simulink model "ravvenController"  (R2018b)
settings: Solver=FixedStepAuto  StartTime=0.0  StopTime=inf  FixedStep=1/1000  RelTol=1e-3  EnableMultiTasking=on
values from neighbouring files (symbols this model uses):
  fs = 1000    [setup.m]
  Ka = [ 4  4   2 ]    [setup.m]
  Kcfa = 0.01    [setup.m]
  Kcfw = 0.99    [setup.m]
  Khd = .3    (= 0.3)    [setup.m]
  Kmixing = [  1   1   1  -1 ... (first row only)    [setup.m]
  Kw = [ .01   .01    .2  ]    [setup.m]
  UseSmallAngleApprox = 0    [setup.m]
  UseTrueThetaPhi = 0    [setup.m]
  w_cmd_lim = 200    [setup.m]
libraries: simulink x6
settings Model: SimulationMode=external  TunableVars=Ka,Kpos,Kvel,Kw  TunableVarsStorageClass=Auto,Auto,Auto,Auto  TunableVarsTypeQualifier=,,,  Creator=kowens  LastModifiedBy=axk1188
settings SolverCC: PositivePriorityOrder=on  AutoInsertRateTranBlk=on
settings DataIOCC: LimitDataPoints=on  SaveFormat=Array  SignalLoggingSaveFormat=ModelDataLogs
settings OptimizationCC: PassReuseOutputArgsAs=Individual arguments  ExpressionDepthLimit=2147483647  MaxStackSize=64
settings DebuggingCC: UnderspecifiedInitializationDetection=Classic  MergeDetectMultiDrivingBlocksExec=none  SolverPrmCheckMsg=warning  ParameterTunabilityLossMsg=error  FcnCallInpInsideContextMsg=warning  StateNameClashWarn=warning  SFUnexpectedBacktrackingDiag=warning  SFNoUnconditionalDefaultTransitionDiag=warning  SFExecutionAtInitializationDiag=none
settings HardwareCC: ProdBitPerPointer=32  ProdBitPerSizeT=32  ProdBitPerPtrDiffT=32  ProdLargestAtomicInteger=Long  ProdLargestAtomicFloat=Double  ProdWordSize=32  ProdHWDeviceType=ARM Compatible->ARM Cortex
settings ModelReferenceCC: PropagateSignalLabelsOutOfModel=off
settings SFSimCC: SimUseLocalCustomCode=off  MATLABDynamicMemAlloc=off
settings RTWCC: SystemTargetFile=ert.tlc  HardwareBoard=Xilinx Zynq-7000 based board  TLCOptions="-aInlineSetEventsForThisBaseRateFcn=TLC_FALSE -aSuppressMultiTaskScheduler=TLC_FALSE  -aRateBasedStepFcn=0"  TemplateMakefile=ert_default_tmf  GenerateReport=on  RTWUseLocalCustomCode=off  Toolchain=Linaro AArch32 Linux v6.3.1  IncludeHyperlinkInReport=on  LaunchReport=on  GenerateTraceInfo=on  GenerateTraceReport=on  GenerateTraceReportSl=on  GenerateTraceReportSf=on  GenerateTraceReportEml=on
settings CodeAppCC: ForceParamTrailComments=on  IgnoreCustomStorageClasses=off  OperatorAnnotations=on  SimulinkDataObjDesc=on  SFDataObjDesc=on  InsertBlockDesc=on
settings ERTTargetCC: SupportNonInlinedSFcns=on
settings ConfigComp: CovMetricSettings=dw  CovHtmlReporting=on  CovSaveCumulativeToWorkspaceVar=on  CovSaveSingleToWorkspaceVar=on  CovExternalEMLEnable=off

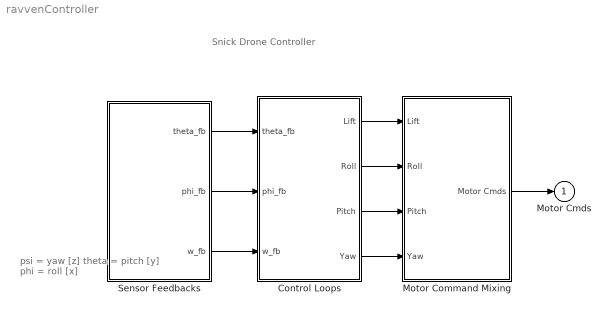
== system ravvenController ==
  note: Snick Drone Controller
  note: psi    =  yaw [z]
      | theta = pitch [y]
      | phi    =  roll [x]
  Control Loops : Subsystem
  Motor Command Mixing : Subsystem
  Sensor Feedbacks : Subsystem
  Motor Cmds : Outport
  wires:
  Control Loops/2(Roll) -> Motor Command Mixing/2(Roll)
  Motor Command Mixing/1(Motor Cmds) -> Motor Cmds/1
  Sensor Feedbacks/2(phi_fb) -> Control Loops/2(phi_fb)
  Control Loops/1(Lift) -> Motor Command Mixing/1(Lift)
  Sensor Feedbacks/3(w_fb) -> Control Loops/3(w_fb)
  Control Loops/4(Yaw) -> Motor Command Mixing/4(Yaw)
  Sensor Feedbacks/1(theta_fb) -> Control Loops/1(theta_fb)
  Control Loops/3(Pitch) -> Motor Command Mixing/3(Pitch)

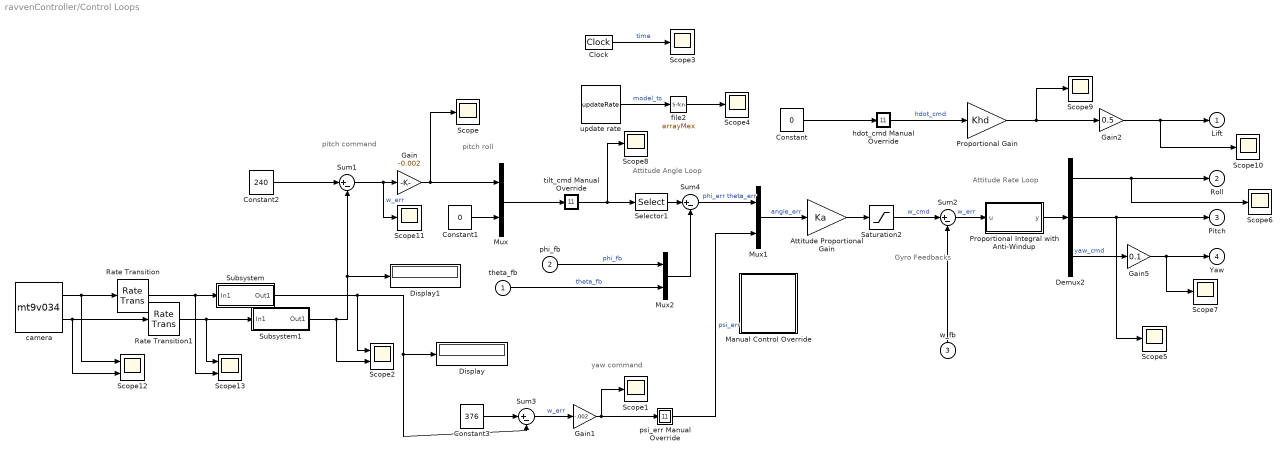
== system ravvenController/Control Loops ==
  note: pitch command
  note: pitch
      | roll
  note: Gyro
      | Feedbacks
  note: Attitude Rate Loop
  note: Attitude Angle Loop
  note: yaw command
  theta_fb : Inport
  phi_fb : Inport  Port=2
  w_fb : Inport  Port=3
  Attitude Proportional Gain : Gain  Gain=Ka
  Clock : DigitalClock  SampleTime=1/fs
  Constant : Constant  Value=0  SampleTime=-1
  Constant1 : Constant  Value=0  SampleTime=1/fs
  Constant2 : Constant  Value=240  SampleTime=1/fs
  Constant3 : Constant  Value=376  SampleTime=1/fs
  Demux2 : Demux  Outputs=3
      settings: AttributesFormatString=%<Outputs>
  Display : Display
  Display1 : Display
  Gain : Gain  Gain=-0.002
  Gain1 : Gain  Gain=-.002
  Gain2 : Gain  Gain=0.5
  Gain5 : Gain  Gain=0.1
  Manual Control Override : Subsystem
      mask Display: disp('Manual\nControl\nOverride')
  Mux : Mux  Inputs=2
  Mux1 : Mux  Inputs=[2 1]
      settings: AttributesFormatString=%<Inputs>
  Mux2 : Mux  Inputs=2
      settings: AttributesFormatString=%<Inputs>
  Proportional Gain : Gain  Gain=Khd
  "Proportional Integral with Anti-Windup " : Subsystem
      mask Display: disp('Kw + Kwi/s')
  Rate Transition : RateTransition  OutPortSampleTime=1/fs
  Rate Transition1 : RateTransition  OutPortSampleTime=1/fs
  Saturation2 : Saturate  UpperLimit=w_cmd_lim  LowerLimit=-w_cmd_lim
      settings: AttributesFormatString=±%<UpperLimit>
  Scope{,1,3..11} (11 alike) : Scope
  Scope12 : Scope  NumInputPorts=2
  Scope13 : Scope  NumInputPorts=2
  Scope2 : Scope  NumInputPorts=2
  Selector1 : Selector  InputPortWidth=2  IndexOptions=Index vector (dialog)  Indices=[2,1]  OutputSizes=1
  Subsystem : Subsystem
  Subsystem1 : Subsystem
  Sum{1..4} (4 alike) : Sum  Inputs=|+-
  "camera " : S-Function  FunctionName=mt9v034  SFunctionDeploymentMode=off  EnableBusSupport=off
      mask Display: image('camera.png');
  file2 : S-Function  FunctionName=arrayMex  Parameters=param1  SFunctionDeploymentMode=off  EnableBusSupport=off  mask{param1=0}
      mask prompts: param1 "File Index"
      mask Display: image('fileImage.png');
  hdot_cmd Manual Override : Subsystem
  psi_err Manual Override : Subsystem
  "tilt_cmd Manual Override " : Subsystem
  update rate : S-Function  FunctionName=updateRate  SFunctionDeploymentMode=off  EnableBusSupport=off
      mask Display: image('clock.png');
  Lift : Outport
  Roll : Outport  Port=2
  Pitch : Outport  Port=3
  Yaw : Outport  Port=4
  wires:
  Selector1/1 -> Sum4/1
  Saturation2/1 -> Sum2/1  "w_cmd"
  Attitude Proportional Gain/1 -> Saturation2/1
  Sum2/1 -> "Proportional Integral with Anti-Windup "/1(u)  "w_err"
  Mux1/1 -> Attitude Proportional Gain/1  "angle_err"
  w_fb/1 -> Sum2/2
  Mux2/1 -> Sum4/2
  Sum4/1 -> Mux1/1  "phi_err theta_err"
  "Proportional Integral with Anti-Windup "/1(y) -> Demux2/1
  phi_fb/1 -> Mux2/1  "phi_fb"
  theta_fb/1 -> Mux2/2  "theta_fb"
  Gain1/1 -> Scope1/1, psi_err Manual Override/1(" ")
  hdot_cmd Manual Override/1(psi_err1) -> Proportional Gain/1  "hdot_cmd"
  "tilt_cmd Manual Override "/1(psi_err1) -> Scope8/1, Selector1/1
  psi_err Manual Override/1(psi_err1) -> Mux1/2  "psi_err"
  Constant1/1 -> Mux/2
  Sum1/1 -> Scope11/1, Gain/1  "w_err"
  Constant2/1 -> Sum1/1
  Gain/1 -> Scope/1, Mux/1
  Constant3/1 -> Sum3/1
  Sum3/1 -> Gain1/1  "w_err"
  Rate Transition/1 -> Scope13/2, Subsystem/1(In1)
  Rate Transition1/1 -> Scope13/1, Subsystem1/1(In1)
  "camera "/1 -> Scope12/1, Rate Transition/1
  "camera "/2 -> Scope12/2, Rate Transition1/1
  Subsystem/1(Out1) -> Scope2/1, Display/1, Sum3/2
  Subsystem1/1(Out1) -> Scope2/2, Display1/1, Sum1/2
  Clock/1 -> Scope3/1  "time"
  update rate/1 -> file2/1  "model_ts"
  Constant/1 -> hdot_cmd Manual Override/1(" ")
  file2/1 -> Scope4/1
  Mux/1 -> "tilt_cmd Manual Override "/1(" ")
  Demux2/3 -> Gain5/1  "yaw_cmd"
  Gain5/1 -> Scope7/1, Yaw/1
  Proportional Gain/1 -> Gain2/1, Scope9/1
  Demux2/1 -> Scope6/1, Roll/1
  Gain2/1 -> Lift/1, Scope10/1
  Demux2/2 -> Pitch/1, Scope5/1

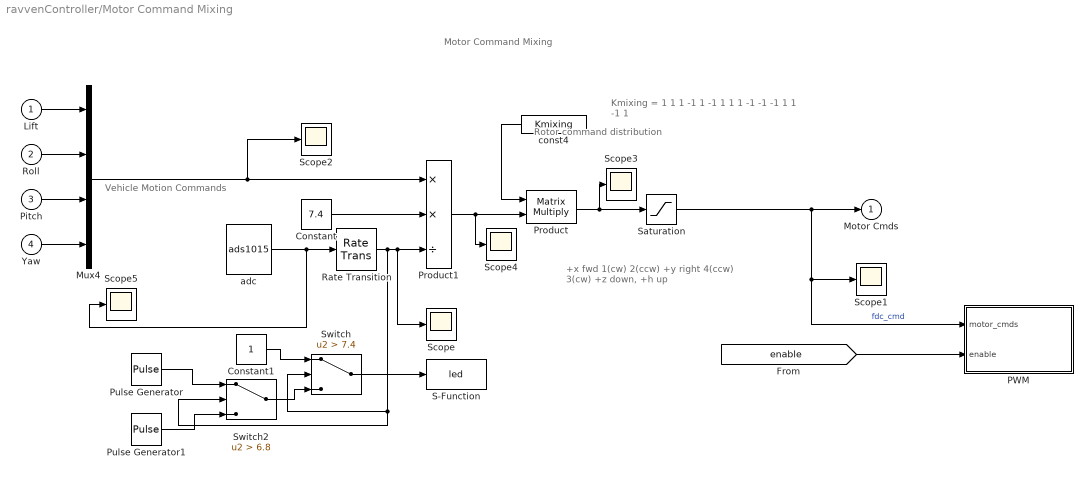
== system ravvenController/Motor Command Mixing ==
  note: Vehicle
      | Motion
      | Commands
  note: +x fwd
      |
      | 1(cw)   2(ccw)
      |                 +y right
      | 4(ccw)   3(cw)
      |
      |    +z down, +h up
  note: Rotor
      | command
      | distribution
  note: Kmixing =
      |      1     1     1    -1
      |      1    -1     1     1
      |      1    -1    -1    -1
      |      1     1    -1     1
  note: Motor Command Mixing
  Lift : Inport
  Roll : Inport  Port=2
  Pitch : Inport  Port=3
  Yaw : Inport  Port=4
  Constant : Constant  Value=7.4  SampleTime=1/fs
  Constant1 : Constant  SampleTime=1/fs
  Mux4 : Mux
      settings: AttributesFormatString=%<Inputs>
  PWM : Subsystem
  Product : Product  Multiplication=Matrix(*)  RndMeth=Zero
  Product1 : Product  Inputs=**/
  Pulse Generator : DiscretePulseGenerator  PulseType=Time based  Period=1  PulseWidth=50
  Pulse Generator1 : DiscretePulseGenerator  PulseType=Time based  Period=0.2  PulseWidth=50
  Rate Transition : RateTransition  OutPortSampleTime=1/fs
  S-Function : S-Function  FunctionName=led  SFunctionDeploymentMode=off  EnableBusSupport=off
  Saturation : Saturate  UpperLimit=1  LowerLimit=0
      settings: AttributesFormatString=%<LowerLimit> - %<UpperLimit>
  Scope{,1..5} (6 alike) : Scope
  Switch : Switch  Criteria=u2 > Threshold  Threshold=7.4
  Switch2 : Switch  Criteria=u2 > Threshold  Threshold=6.8
  adc : S-Function  FunctionName=ads1015  SFunctionDeploymentMode=off  EnableBusSupport=off
      mask Display: image('adc.png');
  const4 : Constant  Value=Kmixing  SampleTime=1/fs
  Motor Cmds : Outport
  wires:
  Yaw/1 -> Mux4/4
  Pitch/1 -> Mux4/3
  Roll/1 -> Mux4/2
  Lift/1 -> Mux4/1
  Saturation/1 -> Scope1/1, PWM/1(motor_cmds), Motor Cmds/1  "fdc_cmd"
  Product/1 -> Scope3/1, Saturation/1
  const4/1 -> Product/1
  [enable] -> PWM/2(enable)
  Product1/1 -> Scope4/1, Product/2
  Mux4/1 -> Scope2/1, Product1/1
  Constant/1 -> Product1/2
  adc/1 -> Scope5/1, Rate Transition/1
  Rate Transition/1 -> Product1/3, Scope/1, Switch2/2, Switch/2
  Constant1/1 -> Switch/1
  Switch2/1 -> Switch/3
  Pulse Generator/1 -> Switch2/1
  Pulse Generator1/1 -> Switch2/3
  Switch/1 -> S-Function/1

== system ravvenController/Sensor Feedbacks ==
  note: Sensor Feedbacks
  note: Acceleration
      | feedbacks
      | (not used)
  Angle Estimation : Subsystem
  IMU : Subsystem
  Terminator_1 : Terminator
  theta_fb : Outport
  phi_fb : Outport  Port=2
  w_fb : Outport  Port=3
  wires:
  IMU/1(wx wy wz) -> w_fb/1, Angle Estimation/2(w_fb)  "w_fb"
  IMU/2("x_accel y_accel z_accel ") -> Angle Estimation/1(a_fb), Terminator_1/1  "a_fb"
  [imu_calibrate] -> IMU/1("imu_calibrate ")
  Angle Estimation/2(phi_est) -> phi_fb/1  "phi_fb_imu"
  Angle Estimation/1(theta_est) -> theta_fb/1  "theta_fb_imu"

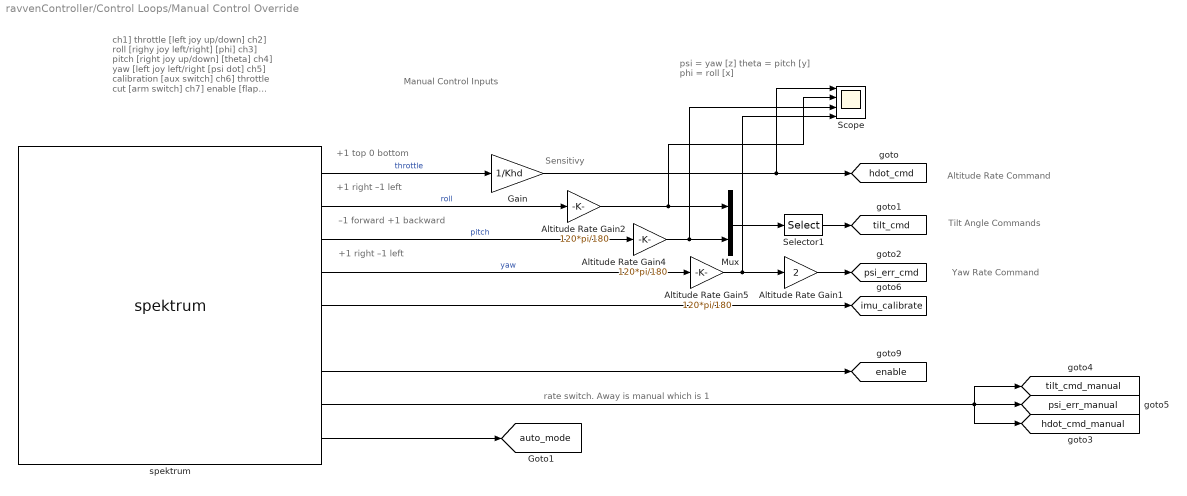
== system ravvenController/Control Loops/Manual Control Override ==
  note: Manual Control Inputs
  note: ch1] throttle [left joy up/down]
      | ch2] roll [righy joy left/right] [phi]
      | ch3] pitch [right joy up/down] [theta]
      | ch4] yaw [left joy left/right [psi dot]
      | ch5] calibration [aux switch]
      | ch6] throttle cut [arm switch]
      | ch7] enable [flap switch]
      | ch8] autonomous [rate switch]
      | ch9] injection [fm switch]
  note: +1 right
      | –1 left
  note: –1 forward
      | +1 backward
  note: +1 right
      | –1 left
  note: +1 top
      | 0 bottom
  note: Yaw Rate Command
  note: Tilt Angle Commands
  note: Altitude Rate Command
  note: Sensitivy
  note: psi    =  yaw [z]
      | theta = pitch [y]
      | phi    =  roll [x]
  note: rate switch. Away is manual which is 1
  Altitude Rate Gain1 : Gain  Gain=2
      settings: AttributesFormatString=%<Gain>
  Altitude Rate Gain2 : Gain  Gain=120*pi/180
      settings: AttributesFormatString=%<Gain>
  Altitude Rate Gain4 : Gain  Gain=120*pi/180
      settings: AttributesFormatString=%<Gain>
  Altitude Rate Gain5 : Gain  Gain=120*pi/180
      settings: AttributesFormatString=%<Gain>
  Gain : Gain  Gain=1/Khd
  Mux : Mux  Inputs=2
  Scope : Scope  NumInputPorts=4
  Selector1 : Selector  InputPortWidth=2  IndexOptions=Index vector (dialog)  Indices=[2,1]  OutputSizes=1
  spektrum : S-Function  FunctionName=spektrum  SFunctionDeploymentMode=off  EnableBusSupport=off
      mask Display: image('spektrum.jpg');
  tag scope: auto_mode=global, enable=global, hdot_cmd=global, hdot_cmd_manual=global, imu_calibrate=global, psi_err_cmd=global, psi_err_manual=global, tilt_cmd=global, tilt_cmd_manual=global
  wires:
  Mux/1 -> Selector1/1
  spektrum/5 -> [imu_calibrate]
  spektrum/1 -> Gain/1  "throttle"
  spektrum/4 -> Altitude Rate Gain5/1  "yaw"
  Gain/1 -> Scope/1, [hdot_cmd]
  spektrum/2 -> Altitude Rate Gain2/1  "roll"
  spektrum/3 -> Altitude Rate Gain4/1  "pitch"
  Altitude Rate Gain2/1 -> Scope/2, Mux/1
  Altitude Rate Gain4/1 -> Scope/3, Mux/2
  Selector1/1 -> [tilt_cmd]
  Altitude Rate Gain5/1 -> Scope/4, Altitude Rate Gain1/1
  Altitude Rate Gain1/1 -> [psi_err_cmd]
  spektrum/7 -> [enable]
  spektrum/8 -> [hdot_cmd_manual], [tilt_cmd_manual], [psi_err_manual]
  spektrum/9 -> [auto_mode]

== system ravvenController/Control Loops/Proportional Integral with Anti-Windup  ==
  note: Proportion Integral with Anti-windup
  note: Discrete Implementation
  u : Inport
  Altitude Integral Gain : Gain  Gain=Kwi./(Kw+(Kw==0))
      settings: AttributesFormatString=%<Gain>
  Rate Proportional Gain : Gain  Gain=Kw
  Saturation2 : Saturate  UpperLimit=1  LowerLimit=-1
      settings: AttributesFormatString=%<LowerLimit> to %<UpperLimit>
  Sum1 : Sum  Inputs=+|-  SaturateOnIntegerOverflow=on  InputSameDT=on  OutDataTypeStr=Inherit: Same as first input
  Sum10 : Sum  Inputs=|++
  Sum5 : Sum  Inputs=|++
  Unit Delay : UnitDelay  SampleTime=-1
      settings: AttributesFormatString=i.c.=%<X0>
  gain2 : Gain  Gain=1/fs
  y : Outport
  wires:
  u/1 -> Rate Proportional Gain/1
  Saturation2/1 -> Sum1/1, y/1
  Altitude Integral Gain/1 -> gain2/1
  Sum1/1 -> Altitude Integral Gain/1
  Sum5/1 -> Saturation2/1
  Rate Proportional Gain/1 -> Sum5/1
  gain2/1 -> Sum10/1
  Sum10/1 -> Unit Delay/1
  Unit Delay/1 -> Sum5/2, Sum1/2, Sum10/2

== system ravvenController/Control Loops/Subsystem ==
  In1 : Inport
  Constant2 : Constant  Value=752  SampleTime=1/fs
  Constant3 : Constant  Value=0  SampleTime=1/fs
  Saturation Dynamic : simulink/Discontinuities/Saturation Dynamic  OutMin=[]  OutMax=[]  OutDataTypeStr=Inherit: Same as second input  OutDataType=fixdt(1, 16)  OutScaling=2^-10  DoSatur=off
  Out1 : Outport
  wires:
  Saturation Dynamic/1 -> Out1/1
  Constant3/1 -> Saturation Dynamic/3
  In1/1 -> Saturation Dynamic/2
  Constant2/1 -> Saturation Dynamic/1

== system ravvenController/Control Loops/Subsystem1 ==
  In1 : Inport
  Constant2 : Constant  Value=480  SampleTime=1/fs
  Constant3 : Constant  Value=0  SampleTime=1/fs
  Saturation Dynamic : simulink/Discontinuities/Saturation Dynamic  OutMin=[]  OutMax=[]  OutDataTypeStr=Inherit: Same as second input  OutDataType=fixdt(1, 16)  OutScaling=2^-10  DoSatur=off
  Out1 : Outport
  wires:
  Constant2/1 -> Saturation Dynamic/1
  In1/1 -> Saturation Dynamic/2
  Constant3/1 -> Saturation Dynamic/3
  Saturation Dynamic/1 -> Out1/1

== system ravvenController/Control Loops/hdot_cmd Manual Override ==
  note: Manual Control
  " " : Inport
  Switch2 : Switch  Threshold=0.5
  psi_err1 : Outport
  wires:
  [hdot_cmd_manual] -> Switch2/2
  [hdot_cmd] -> Switch2/3, Switch2/1
  Switch2/1 -> psi_err1/1

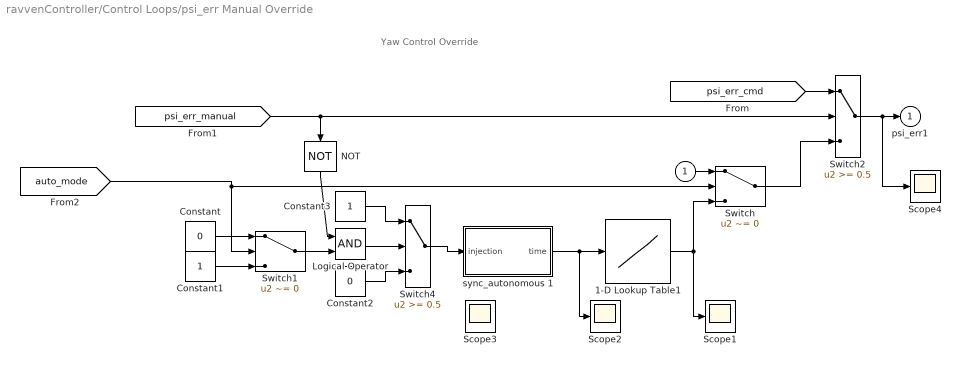
== system ravvenController/Control Loops/psi_err Manual Override ==
  note: Yaw Control Override
  " " : Inport
  1-D Lookup Table1 : Lookup_n-D  NumberOfTableDimensions=1  BreakpointsForDimension1=[0,3,6,9,12,15,18,21,24]  Table=[0,0,0,0,0,1.5708,0,-1.5708,0]  InterpMethod=Flat  ExtrapMethod=Cubic spline  UseLastTableValue=on  InternalRulePriority=Speed  RndMeth=Simplest  InputSameDT=on
  Constant : Constant  Value=0  SampleTime=-1
  Constant1 : Constant  SampleTime=-1
  Constant2 : Constant  Value=0  SampleTime=-1
  Constant3 : Constant  SampleTime=-1
  Logical Operator : Logic  AllPortsSameDT=off  OutDataTypeStr=boolean
  NOT : Logic  Operator=NOT  IconShape=distinctive  AllPortsSameDT=off  OutDataTypeStr=boolean
  Scope{1..4} (4 alike) : Scope
  Switch : Switch  Criteria=u2 ~= 0
  Switch1 : Switch  Criteria=u2 ~= 0
  Switch2 : Switch  Threshold=0.5
  Switch4 : Switch  Threshold=0.5
  sync_autonomous 1 : Subsystem
  psi_err1 : Outport
  wires:
  Switch2/1 -> Scope4/1, psi_err1/1
  [psi_err_cmd] -> Switch2/1
  Switch/1 -> Switch2/3
  [auto_mode] -> Switch1/2, Switch/2
  Constant/1 -> Switch1/1
  Constant1/1 -> Switch1/3
  sync_autonomous 1/1("time ") -> Scope2/1, 1-D Lookup Table1/1
  " "/1 -> Switch/1
  1-D Lookup Table1/1 -> Scope1/1, Switch/3
  [psi_err_manual] -> NOT/1, Switch2/2
  Switch4/1 -> sync_autonomous 1/1("injection ")
  NOT/1 -> Logical Operator/1
  Logical Operator/1 -> Switch4/2
  Switch1/1 -> Logical Operator/2
  Constant3/1 -> Switch4/1
  Constant2/1 -> Switch4/3

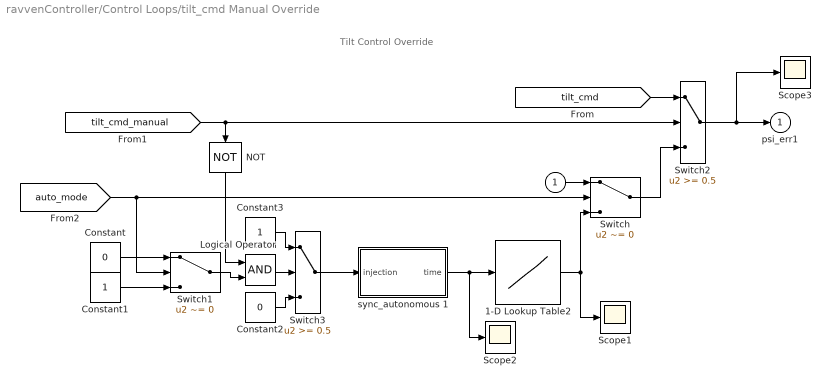
== system ravvenController/Control Loops/tilt_cmd Manual Override  ==
  note: Tilt Control Override
  " " : Inport
  1-D Lookup Table2 : Lookup_n-D  NumberOfTableDimensions=1  BreakpointsForDimension1=[0,3,6,9,12,15,18,21,24]  Table=[0,0.523599,0,-0.523599,0,0,0,0,0]  InterpMethod=Flat  InternalRulePriority=Speed  RndMeth=Simplest  InputSameDT=on
  Constant : Constant  Value=0  SampleTime=-1
  Constant1 : Constant  SampleTime=-1
  Constant2 : Constant  Value=0  SampleTime=-1
  Constant3 : Constant  SampleTime=-1
  Logical Operator : Logic  AllPortsSameDT=off  OutDataTypeStr=boolean
  NOT : Logic  Operator=NOT  IconShape=distinctive  AllPortsSameDT=off  OutDataTypeStr=boolean
  Scope1 : Scope
  Scope2 : Scope
  Scope3 : Scope
  Switch : Switch  Criteria=u2 ~= 0
  Switch1 : Switch  Criteria=u2 ~= 0
  Switch2 : Switch  Threshold=0.5
  Switch3 : Switch  Threshold=0.5
  sync_autonomous 1 : Subsystem
  psi_err1 : Outport
  wires:
  [tilt_cmd] -> Switch2/1
  Switch2/1 -> Scope3/1, psi_err1/1
  sync_autonomous 1/1("time ") -> Scope2/1, 1-D Lookup Table2/1
  Constant1/1 -> Switch1/3
  [auto_mode] -> Switch1/2, Switch/2
  Constant/1 -> Switch1/1
  1-D Lookup Table2/1 -> Switch/3, Scope1/1
  Switch/1 -> Switch2/3
  [tilt_cmd_manual] -> Switch2/2, NOT/1
  " "/1 -> Switch/1
  Switch1/1 -> Logical Operator/2
  Switch3/1 -> sync_autonomous 1/1("injection ")
  Logical Operator/1 -> Switch3/2
  NOT/1 -> Logical Operator/1
  Constant2/1 -> Switch3/3
  Constant3/1 -> Switch3/1

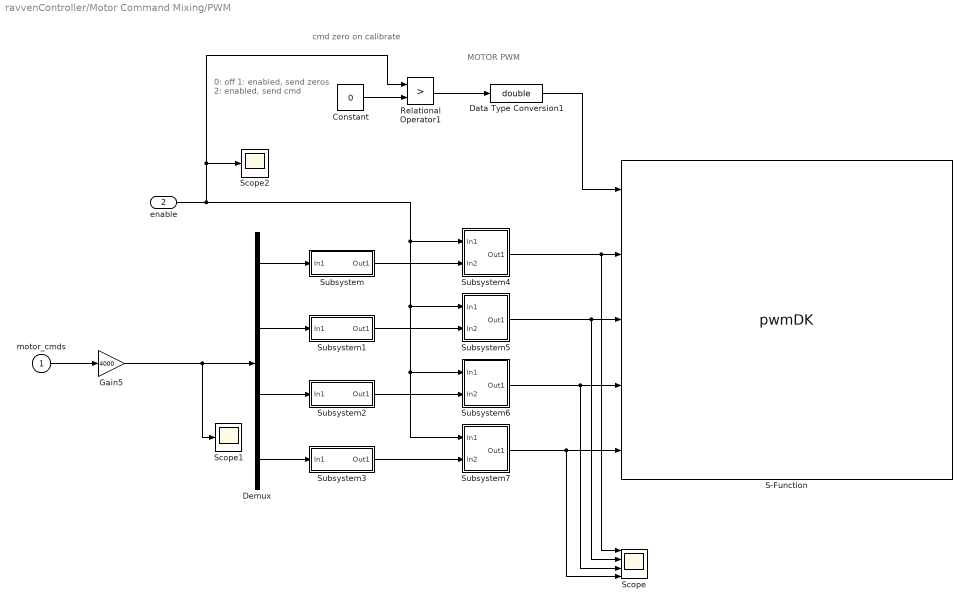
== system ravvenController/Motor Command Mixing/PWM ==
  note: 0: off
      | 1: enabled, send zeros
      | 2: enabled, send cmd
  note: cmd zero on calibrate
  note: MOTOR PWM
  motor_cmds : Inport
  enable : Inport  Port=2
  Constant : Constant  Value=0  SampleTime=1/fs
  Data Type Conversion1 : DataTypeConversion  OutDataTypeStr=double
  Demux : Demux
  Gain5 : Gain  Gain=4000
  Relational Operator1 : RelationalOperator  Operator=>  RndMeth=Simplest
  S-Function : S-Function  FunctionName=pwmDK  SFunctionDeploymentMode=off  EnableBusSupport=off
      mask Display: image('pwm.jpg');
  Scope : Scope  NumInputPorts=4
  Scope1 : Scope
  Scope2 : Scope
  Subsystem : Subsystem
  Subsystem1 : Subsystem
  Subsystem2 : Subsystem
  Subsystem3 : Subsystem
  Subsystem4 : Subsystem
  Subsystem5 : Subsystem
  Subsystem6 : Subsystem
  Subsystem7 : Subsystem
  wires:
  motor_cmds/1 -> Gain5/1
  Relational Operator1/1 -> Data Type Conversion1/1
  Constant/1 -> Relational Operator1/2
  Data Type Conversion1/1 -> S-Function/1
  Demux/1 -> Subsystem/1(In1)
  Demux/2 -> Subsystem1/1(In1)
  Demux/3 -> Subsystem2/1(In1)
  Demux/4 -> Subsystem3/1(In1)
  enable/1 -> Subsystem5/1(In1), Subsystem7/1(In1), Subsystem6/1(In1), Subsystem4/1(In1), Relational Operator1/1, Scope2/1
  Subsystem/1(Out1) -> Subsystem4/2(In2)
  Subsystem1/1(Out1) -> Subsystem5/2(In2)
  Subsystem2/1(Out1) -> Subsystem6/2(In2)
  Subsystem3/1(Out1) -> Subsystem7/2(In2)
  Gain5/1 -> Scope1/1, Demux/1
  Subsystem4/1(Out1) -> Scope/1, S-Function/2
  Subsystem5/1(Out1) -> Scope/2, S-Function/3
  Subsystem6/1(Out1) -> Scope/3, S-Function/4
  Subsystem7/1(Out1) -> Scope/4, S-Function/5

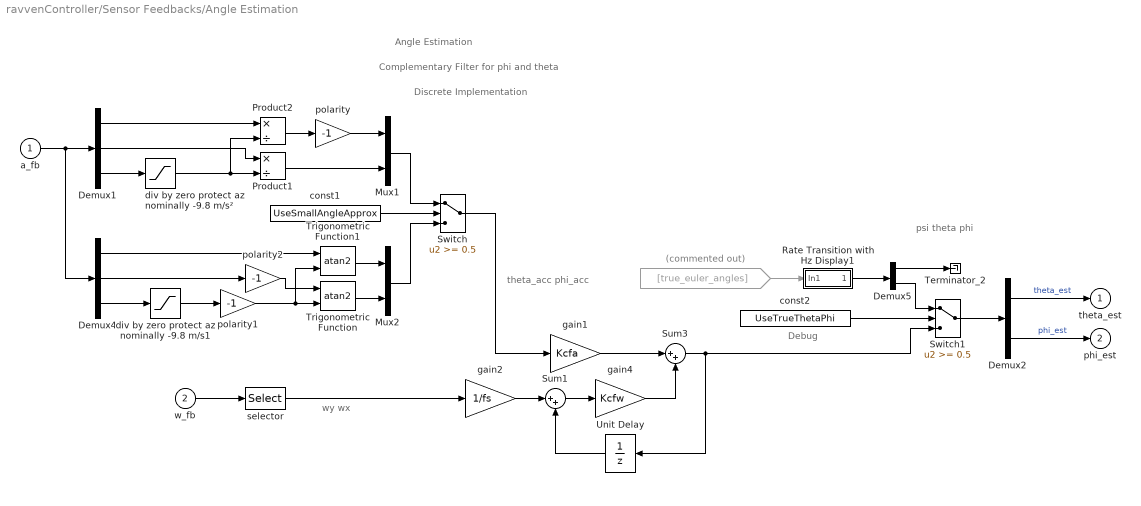
== system ravvenController/Sensor Feedbacks/Angle Estimation ==
  note: Debug
  note: psi
      | theta
      | phi
  note: theta_acc
      | phi_acc
  note: wy
      | wx
  note: Discrete Implementation
  note: Complementary Filter for phi and theta
  note: Angle Estimation
  a_fb : Inport
  w_fb : Inport  Port=2
  " " : From  Commented=on  GotoTag=true_euler_angles  TagVisibility=global
  Demux1 : Demux  Outputs=3
      settings: AttributesFormatString=%<Outputs>
  Demux2 : Demux  Outputs=[1 1]
      settings: AttributesFormatString=%<Outputs>
  Demux4 : Demux  Outputs=3
      settings: AttributesFormatString=%<Outputs>
  Demux5 : Demux  Outputs=[1 2]
      settings: AttributesFormatString=%<Outputs>
  Mux1 : Mux  Inputs=2
      settings: AttributesFormatString=%<Inputs>
  Mux2 : Mux  Inputs=2
      settings: AttributesFormatString=%<Inputs>
  Product1 : Product  Inputs=*/  RndMeth=Zero
  Product2 : Product  Inputs=*/  RndMeth=Zero
  Rate Transition with Hz Display1 : Subsystem  mask(Rate Transition with Hz Display){f=fs, ic=0}
      mask prompts: f "Update Frequency"; ic "Initial Conditions"
      mask init:
      | if isinf(f)
      |   sss='cont';
      | elseif f==0
      |   sss='cont';
      | elseif f>1e9
      |   sss=[num2str(f/1e9) ' GHz'];
      | elseif f>1e6
      |   sss=[num2str(f/1e6) ' MHz'];
      | elseif f>1e3
      |   sss=[num2str(f/1e3) ' kHz'];
      | else
      |   sss=[num2str(f) ' Hz'];
      | end
      | Ts=(f>0)/(f+(f==0));    
      | % 1/f for f>0
      | % 0 for f=0
      mask Display: disp(sss);
  Sum1 : Sum  Inputs=|++
  Sum3 : Sum  Inputs=|++
  Switch : Switch  Threshold=0.5
  Switch1 : Switch  Threshold=0.5
  Terminator_2 : Terminator
  Trigonometric Function : Trigonometry  Operator=atan2
  Trigonometric Function1 : Trigonometry  Operator=atan2
  Unit Delay : UnitDelay  SampleTime=-1
  const1 : Constant  Value=UseSmallAngleApprox
  const2 : Constant  Value=UseTrueThetaPhi
  div by zero protect az nominally -9.8 m/s1 : Saturate  UpperLimit=-1  LowerLimit=-20
      settings: AttributesFormatString=%<LowerLimit> to %<UpperLimit>
  div by zero protect az nominally -9.8 m/s² : Saturate  UpperLimit=-1  LowerLimit=-20
      settings: AttributesFormatString=%<LowerLimit> to %<UpperLimit>
  gain1 : Gain  Gain=Kcfa
  gain2 : Gain  Gain=1/fs
  gain4 : Gain  Gain=Kcfw
  polarity : Gain  Gain=-1
  polarity1 : Gain  Gain=-1
  polarity2 : Gain  Gain=-1
  selector : Selector  InputPortWidth=3  IndexOptions=Index vector (dialog)  Indices=[2,1]  OutputSizes=1
  theta_est : Outport
  phi_est : Outport  Port=2
  wires:
  Rate Transition with Hz Display1/1(Out1) -> Demux5/1
  Demux5/1 -> Terminator_2/1
  Demux5/2 -> Switch1/1
  " "/1 -> Rate Transition with Hz Display1/1(In1)
  Switch1/1 -> Demux2/1
  const2/1 -> Switch1/2
  Switch/1 -> gain1/1
  const1/1 -> Switch/2
  Mux2/1 -> Switch/3
  Mux1/1 -> Switch/1
  polarity2/1 -> Trigonometric Function/1
  Demux4/2 -> polarity2/1
  polarity1/1 -> Trigonometric Function1/2, Trigonometric Function/2
  Trigonometric Function1/1 -> Mux2/1
  Trigonometric Function/1 -> Mux2/2
  Demux4/1 -> Trigonometric Function1/1
  div by zero protect az nominally -9.8 m/s1/1 -> polarity1/1
  Demux4/3 -> div by zero protect az nominally -9.8 m/s1/1
  Product2/1 -> polarity/1
  Demux1/1 -> Product2/1
  selector/1 -> gain2/1
  Demux2/2 -> phi_est/1  "phi_est"
  Demux2/1 -> theta_est/1  "theta_est"
  Sum3/1 -> Unit Delay/1, Switch1/3
  gain2/1 -> Sum1/1
  gain1/1 -> Sum3/1
  gain4/1 -> Sum3/2
  Unit Delay/1 -> Sum1/2
  Sum1/1 -> gain4/1
  Product1/1 -> Mux1/2
  a_fb/1 -> Demux4/1, Demux1/1
  polarity/1 -> Mux1/1
  div by zero protect az nominally -9.8 m/s²/1 -> Product1/2, Product2/2
  Demux1/2 -> Product1/1
  Demux1/3 -> div by zero protect az nominally -9.8 m/s²/1
  w_fb/1 -> selector/1

== system ravvenController/Sensor Feedbacks/IMU ==
  note: gyro in rad/s
  note: accel in m/s^2
  "imu_calibrate " : Inport
  IMU Calibration : Subsystem
  Mux1 : Mux  Inputs=3
  Mux2 : Mux  Inputs=3
  Scope : Scope
  Scope1 : Scope
  mpu9250 : S-Function  FunctionName=mpu9250  SFunctionDeploymentMode=off  EnableBusSupport=off
      mask Display: image('imu.png');
  wx wy wz : Outport
  "x_accel y_accel z_accel " : Outport  Port=2
  wires:
  mpu9250/4 -> Mux2/1
  mpu9250/5 -> Mux2/2
  mpu9250/3 -> Mux1/3
  mpu9250/6 -> Mux2/3
  mpu9250/2 -> Mux1/2
  mpu9250/1 -> Mux1/1
  Mux1/1 -> IMU Calibration/1(a_fb_raw)
  Mux2/1 -> IMU Calibration/2(w_fb_raw)
  IMU Calibration/1(a_fb) -> Scope/1, "x_accel y_accel z_accel "/1
  IMU Calibration/2(w_fb) -> Scope1/1, wx wy wz/1
  "imu_calibrate "/1 -> IMU Calibration/3(imu_calibrate)

== system ravvenController/Control Loops/psi_err Manual Override/sync_autonomous 1 ==
  note: injection = 0 => pass through 0
      | injection = 1 => start clock
  "injection " : Inport
  Bias : Bias  Bias=0.001
  Constant : Constant  Value=0  SampleTime=-1
  Constant1 : Constant  Commented=on  Value=0  SampleTime=-1
  Switch : Switch  Criteria=u2 ~= 0
  Switch1 : Switch  Commented=on  Criteria=u2 > Threshold  Threshold=25
  Unit Delay : UnitDelay  SampleTime=-1
  "time " : Outport
  wires:
  Constant/1 -> Switch/3
  Bias/1 -> Switch/1
  "injection "/1 -> Switch/2
  Unit Delay/1 -> Bias/1
  Switch/1 -> Unit Delay/1, "time "/1
  Constant1/1 -> Switch1/1

== system ravvenController/Control Loops/tilt_cmd Manual Override /sync_autonomous 1 ==
  note: injection = 0 => pass through 0
      | injection = 1 => start clock
  "injection " : Inport
  Bias : Bias  Bias=0.001
  Constant : Constant  Value=0  SampleTime=-1
  Constant1 : Constant  Value=0  SampleTime=-1
  Switch : Switch  Criteria=u2 ~= 0
  Switch1 : Switch  Criteria=u2 > Threshold  Threshold=25
  Unit Delay : UnitDelay  SampleTime=-1
  "time " : Outport
  wires:
  Constant/1 -> Switch/3
  Bias/1 -> Switch/1
  "injection "/1 -> Switch/2
  Unit Delay/1 -> Bias/1
  Switch1/1 -> Unit Delay/1, "time "/1
  Switch/1 -> Switch1/3, Switch1/2
  Constant1/1 -> Switch1/1

== system ravvenController/Motor Command Mixing/PWM/Subsystem ==
  In1 : Inport
  Constant2 : Constant  Value=1700  SampleTime=1/fs
  Constant3 : Constant  Value=100  SampleTime=1/fs
  Saturation Dynamic : simulink/Discontinuities/Saturation Dynamic  OutMin=[]  OutMax=[]  OutDataTypeStr=Inherit: Same as second input  OutDataType=fixdt(1, 16)  OutScaling=2^-10  DoSatur=off
  Scope1 : Scope
  Scope2 : Scope
  Out1 : Outport
  wires:
  Saturation Dynamic/1 -> Scope1/1, Out1/1
  Constant3/1 -> Saturation Dynamic/3
  In1/1 -> Scope2/1, Saturation Dynamic/2
  Constant2/1 -> Saturation Dynamic/1

== system ravvenController/Motor Command Mixing/PWM/Subsystem1 ==
  In1 : Inport
  Constant2 : Constant  Value=1700  SampleTime=1/fs
  Constant3 : Constant  Value=100  SampleTime=1/fs
  Saturation Dynamic : simulink/Discontinuities/Saturation Dynamic  OutMin=[]  OutMax=[]  OutDataTypeStr=Inherit: Same as second input  OutDataType=fixdt(1, 16)  OutScaling=2^-10  DoSatur=off
  Scope1 : Scope
  Scope2 : Scope
  Out1 : Outport
  wires:
  Constant2/1 -> Saturation Dynamic/1
  In1/1 -> Saturation Dynamic/2, Scope2/1
  Constant3/1 -> Saturation Dynamic/3
  Saturation Dynamic/1 -> Out1/1, Scope1/1

== system ravvenController/Motor Command Mixing/PWM/Subsystem2 ==
  In1 : Inport
  Constant2 : Constant  Value=1700  SampleTime=1/fs
  Constant3 : Constant  Value=100  SampleTime=1/fs
  Saturation Dynamic : simulink/Discontinuities/Saturation Dynamic  OutMin=[]  OutMax=[]  OutDataTypeStr=Inherit: Same as second input  OutDataType=fixdt(1, 16)  OutScaling=2^-10  DoSatur=off
  Scope1 : Scope
  Scope2 : Scope
  Out1 : Outport
  wires:
  Saturation Dynamic/1 -> Scope1/1, Out1/1
  Constant3/1 -> Saturation Dynamic/3
  In1/1 -> Scope2/1, Saturation Dynamic/2
  Constant2/1 -> Saturation Dynamic/1

== system ravvenController/Motor Command Mixing/PWM/Subsystem3 ==
  In1 : Inport
  Constant2 : Constant  Value=1700  SampleTime=1/fs
  Constant3 : Constant  Value=100  SampleTime=1/fs
  Saturation Dynamic : simulink/Discontinuities/Saturation Dynamic  OutMin=[]  OutMax=[]  OutDataTypeStr=Inherit: Same as second input  OutDataType=fixdt(1, 16)  OutScaling=2^-10  DoSatur=off
  Scope1 : Scope
  Scope2 : Scope
  Out1 : Outport
  wires:
  Constant2/1 -> Saturation Dynamic/1
  In1/1 -> Saturation Dynamic/2, Scope2/1
  Constant3/1 -> Saturation Dynamic/3
  Saturation Dynamic/1 -> Out1/1, Scope1/1

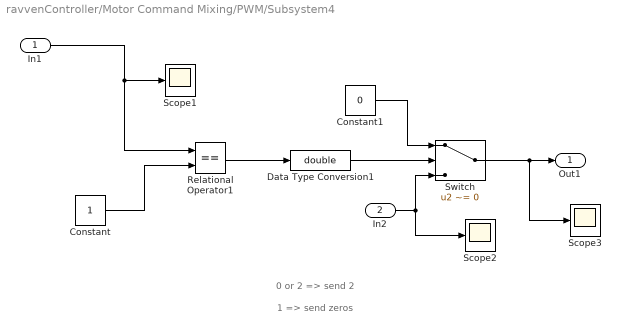
== system ravvenController/Motor Command Mixing/PWM/Subsystem4 ==
  note: 1 => send zeros
  note: 0 or 2 => send 2
  In1 : Inport
  In2 : Inport  Port=2
  Constant : Constant  SampleTime=1/fs
  Constant1 : Constant  Value=0  SampleTime=1/fs
  Data Type Conversion1 : DataTypeConversion  OutDataTypeStr=double
  Relational Operator1 : RelationalOperator  Operator===  RndMeth=Simplest
  Scope1 : Scope
  Scope2 : Scope
  Scope3 : Scope
  Switch : Switch  Criteria=u2 ~= 0  Threshold=1
  Out1 : Outport
  wires:
  Constant/1 -> Relational Operator1/2
  Relational Operator1/1 -> Data Type Conversion1/1
  Data Type Conversion1/1 -> Switch/2
  Switch/1 -> Scope3/1, Out1/1
  In1/1 -> Scope1/1, Relational Operator1/1
  Constant1/1 -> Switch/1
  In2/1 -> Scope2/1, Switch/3

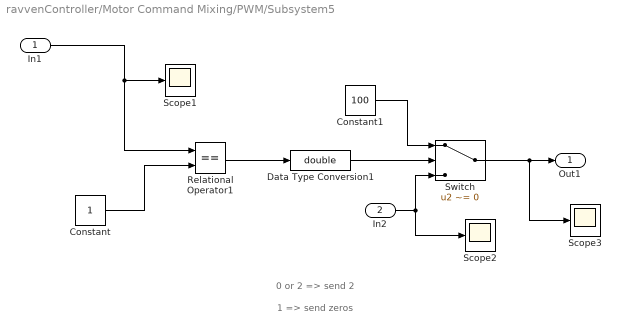
== system ravvenController/Motor Command Mixing/PWM/Subsystem5 ==
  note: 0 or 2 => send 2
  note: 1 => send zeros
  In1 : Inport
  In2 : Inport  Port=2
  Constant : Constant  SampleTime=1/fs
  Constant1 : Constant  Value=100  SampleTime=1/fs
  Data Type Conversion1 : DataTypeConversion  OutDataTypeStr=double
  Relational Operator1 : RelationalOperator  Operator===  RndMeth=Simplest
  Scope1 : Scope
  Scope2 : Scope
  Scope3 : Scope
  Switch : Switch  Criteria=u2 ~= 0  Threshold=1
  Out1 : Outport
  wires:
  In2/1 -> Switch/3, Scope2/1
  Constant1/1 -> Switch/1
  In1/1 -> Relational Operator1/1, Scope1/1
  Switch/1 -> Out1/1, Scope3/1
  Data Type Conversion1/1 -> Switch/2
  Relational Operator1/1 -> Data Type Conversion1/1
  Constant/1 -> Relational Operator1/2

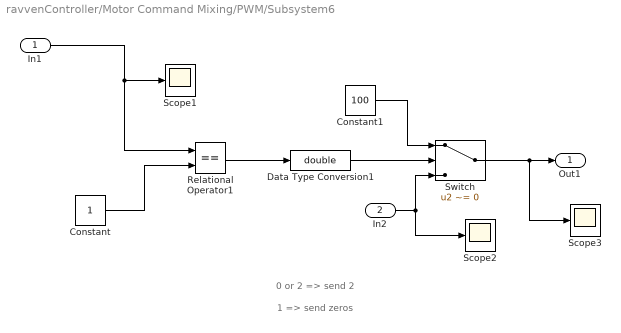
== system ravvenController/Motor Command Mixing/PWM/Subsystem6 ==
  note: 1 => send zeros
  note: 0 or 2 => send 2
  In1 : Inport
  In2 : Inport  Port=2
  Constant : Constant  SampleTime=1/fs
  Constant1 : Constant  Value=100  SampleTime=1/fs
  Data Type Conversion1 : DataTypeConversion  OutDataTypeStr=double
  Relational Operator1 : RelationalOperator  Operator===  RndMeth=Simplest
  Scope1 : Scope
  Scope2 : Scope
  Scope3 : Scope
  Switch : Switch  Criteria=u2 ~= 0  Threshold=1
  Out1 : Outport
  wires:
  Constant/1 -> Relational Operator1/2
  Relational Operator1/1 -> Data Type Conversion1/1
  Data Type Conversion1/1 -> Switch/2
  Switch/1 -> Scope3/1, Out1/1
  In1/1 -> Scope1/1, Relational Operator1/1
  Constant1/1 -> Switch/1
  In2/1 -> Scope2/1, Switch/3

== system ravvenController/Motor Command Mixing/PWM/Subsystem7 ==
  note: 0 or 2 => send 2
  note: 1 => send zeros
  In1 : Inport
  In2 : Inport  Port=2
  Constant : Constant  SampleTime=1/fs
  Constant1 : Constant  Value=100  SampleTime=1/fs
  Data Type Conversion1 : DataTypeConversion  OutDataTypeStr=double
  Relational Operator1 : RelationalOperator  Operator===  RndMeth=Simplest
  Scope1 : Scope
  Scope2 : Scope
  Scope3 : Scope
  Switch : Switch  Criteria=u2 ~= 0  Threshold=1
  Out1 : Outport
  wires:
  In2/1 -> Switch/3, Scope2/1
  Constant1/1 -> Switch/1
  In1/1 -> Relational Operator1/1, Scope1/1
  Switch/1 -> Out1/1, Scope3/1
  Data Type Conversion1/1 -> Switch/2
  Relational Operator1/1 -> Data Type Conversion1/1
  Constant/1 -> Relational Operator1/2

== system ravvenController/Sensor Feedbacks/Angle Estimation/Rate Transition with Hz Display1 ==
  In1 : Inport
  Rate Transition8 : RateTransition  InitialCondition=ic  OutPortSampleTime=Ts
  Out1 : Outport
  wires:
  In1/1 -> Rate Transition8/1
  Rate Transition8/1 -> Out1/1

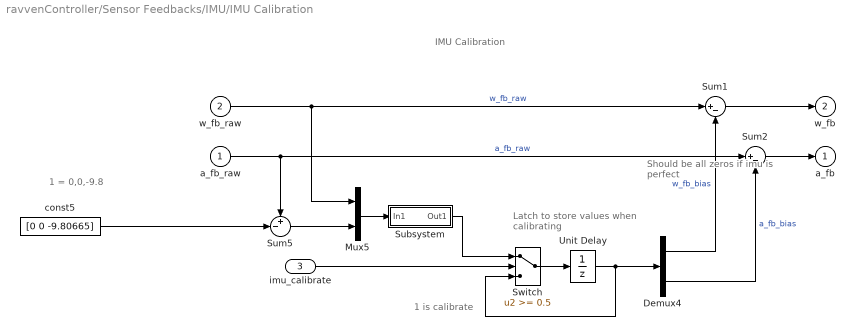
== system ravvenController/Sensor Feedbacks/IMU/IMU Calibration ==
  note: 1 = 0,0,-9.8
  note: 1 is calibrate
  note: IMU Calibration
  note: Latch to store values
      | when calibrating
  note: Should be all
      | zeros if
      | imu is perfect
  a_fb_raw : Inport
  w_fb_raw : Inport  Port=2
  imu_calibrate : Inport  Port=3
  Demux4 : Demux  Outputs=[3 3]
      settings: AttributesFormatString=%<Outputs>
  Mux5 : Mux  Inputs=[3 3]
      settings: AttributesFormatString=%<Inputs>
  Subsystem : Subsystem
  Sum1 : Sum  Inputs=|+-
  Sum2 : Sum  Inputs=|+-
  Sum5 : Sum  Inputs=+-|
  Switch : Switch  Threshold=0.5
  Unit Delay : UnitDelay  InitialCondition=[0 0 0 0 0 0]  SampleTime=-1
  const5 : Constant  Value=[0 0 -9.80665]  SampleTime=1/fs
  a_fb : Outport
  w_fb : Outport  Port=2
  wires:
  w_fb_raw/1 -> Sum1/1, Mux5/1  "w_fb_raw"
  a_fb_raw/1 -> Sum2/1, Sum5/1  "a_fb_raw"
  Sum1/1 -> w_fb/1
  Sum2/1 -> a_fb/1
  Switch/1 -> Unit Delay/1
  Demux4/1 -> Sum1/2  "w_fb_bias"
  Demux4/2 -> Sum2/2  "a_fb_bias"
  Unit Delay/1 -> Switch/3, Demux4/1
  Sum5/1 -> Mux5/2
  Mux5/1 -> Subsystem/1(In1)
  Subsystem/1(Out1) -> Switch/1
  imu_calibrate/1 -> Switch/2
  const5/1 -> Sum5/2

== system ravvenController/Sensor Feedbacks/IMU/IMU Calibration/Subsystem ==
  In1 : Inport
  Demux : Demux  Outputs=6
  Mux : Mux  Inputs=6
  Subsystem1 : Subsystem
  Subsystem2 : Subsystem
  Subsystem3 : Subsystem
  Subsystem4 : Subsystem
  Subsystem5 : Subsystem
  Subsystem6 : Subsystem
  Out1 : Outport
  wires:
  In1/1 -> Demux/1
  Mux/1 -> Out1/1
  Demux/1 -> Subsystem5/1(In1)
  Demux/2 -> Subsystem1/1(In1)
  Demux/3 -> Subsystem2/1(In1)
  Demux/4 -> Subsystem6/1(In1)
  Demux/5 -> Subsystem3/1(In1)
  Demux/6 -> Subsystem4/1(In1)
  Subsystem5/1(Out1) -> Mux/1
  Subsystem1/1(Out1) -> Mux/2
  Subsystem2/1(Out1) -> Mux/3
  Subsystem6/1(Out1) -> Mux/4
  Subsystem3/1(Out1) -> Mux/5
  Subsystem4/1(Out1) -> Mux/6

== system ravvenController/Sensor Feedbacks/IMU/IMU Calibration/Subsystem/Subsystem1 ==
  In1 : Inport
  Demux : Demux  Outputs=[9 1]
  Gain : Gain  Gain=.1
  Mux : Mux  Inputs=[1 9]
  Sum : Sum  Inputs=+
  Terminator : Terminator
  Unit Delay : UnitDelay  SampleTime=-1
  Out1 : Outport
  wires:
  Gain/1 -> Out1/1
  Sum/1 -> Gain/1
  Demux/2 -> Terminator/1
  Mux/1 -> Unit Delay/1, Sum/1
  In1/1 -> Mux/1
  Demux/1 -> Mux/2
  Unit Delay/1 -> Demux/1

== system ravvenController/Sensor Feedbacks/IMU/IMU Calibration/Subsystem/Subsystem2 ==
  In1 : Inport
  Demux : Demux  Outputs=[9 1]
  Gain : Gain  Gain=.1
  Mux : Mux  Inputs=[1 9]
  Sum : Sum  Inputs=+
  Terminator : Terminator
  Unit Delay : UnitDelay  SampleTime=-1
  Out1 : Outport
  wires:
  Gain/1 -> Out1/1
  Sum/1 -> Gain/1
  Demux/2 -> Terminator/1
  Mux/1 -> Unit Delay/1, Sum/1
  In1/1 -> Mux/1
  Demux/1 -> Mux/2
  Unit Delay/1 -> Demux/1

== system ravvenController/Sensor Feedbacks/IMU/IMU Calibration/Subsystem/Subsystem3 ==
  In1 : Inport
  Demux : Demux  Outputs=[9 1]
  Gain : Gain  Gain=.1
  Mux : Mux  Inputs=[1 9]
  Sum : Sum  Inputs=+
  Terminator : Terminator
  Unit Delay : UnitDelay  SampleTime=-1
  Out1 : Outport
  wires:
  Gain/1 -> Out1/1
  Sum/1 -> Gain/1
  Demux/2 -> Terminator/1
  Mux/1 -> Unit Delay/1, Sum/1
  In1/1 -> Mux/1
  Demux/1 -> Mux/2
  Unit Delay/1 -> Demux/1

== system ravvenController/Sensor Feedbacks/IMU/IMU Calibration/Subsystem/Subsystem4 ==
  In1 : Inport
  Demux : Demux  Outputs=[9 1]
  Gain : Gain  Gain=.1
  Mux : Mux  Inputs=[1 9]
  Sum : Sum  Inputs=+
  Terminator : Terminator
  Unit Delay : UnitDelay  SampleTime=-1
  Out1 : Outport
  wires:
  Gain/1 -> Out1/1
  Sum/1 -> Gain/1
  Demux/2 -> Terminator/1
  Mux/1 -> Unit Delay/1, Sum/1
  In1/1 -> Mux/1
  Demux/1 -> Mux/2
  Unit Delay/1 -> Demux/1

== system ravvenController/Sensor Feedbacks/IMU/IMU Calibration/Subsystem/Subsystem5 ==
  In1 : Inport
  Demux : Demux  Outputs=[9 1]
  Gain : Gain  Gain=.1
  Mux : Mux  Inputs=[1 9]
  Sum : Sum  Inputs=+
  Terminator : Terminator
  Unit Delay : UnitDelay  SampleTime=-1
  Out1 : Outport
  wires:
  Gain/1 -> Out1/1
  Sum/1 -> Gain/1
  Demux/2 -> Terminator/1
  Mux/1 -> Unit Delay/1, Sum/1
  In1/1 -> Mux/1
  Demux/1 -> Mux/2
  Unit Delay/1 -> Demux/1

== system ravvenController/Sensor Feedbacks/IMU/IMU Calibration/Subsystem/Subsystem6 ==
  In1 : Inport
  Demux : Demux  Outputs=[9 1]
  Gain : Gain  Gain=.1
  Mux : Mux  Inputs=[1 9]
  Sum : Sum  Inputs=+
  Terminator : Terminator
  Unit Delay : UnitDelay  SampleTime=-1
  Out1 : Outport
  wires:
  Gain/1 -> Out1/1
  Sum/1 -> Gain/1
  Demux/2 -> Terminator/1
  Mux/1 -> Unit Delay/1, Sum/1
  In1/1 -> Mux/1
  Demux/1 -> Mux/2
  Unit Delay/1 -> Demux/1
